simulink model "coneDetectionWithObjectDetectorBlock"  (R2025a)
settings: Solver=VariableStepAuto  StartTime=0.0  StopTime=50  RelTol=1e-3
undefined symbols (not defined in the file or in its folder): gray
libraries: visionanalysis x1, dspvision x1
settings Model: Creator=gracew  LastModifiedBy=lipingw
settings OptimizationCC: ReuseModelBlockBuffer=off
settings SFSimCC: SimTargetLang=C++  SimDLTargetLibrary=mkl-dnn
settings RTWCC: GPUComputeCapability=3.5

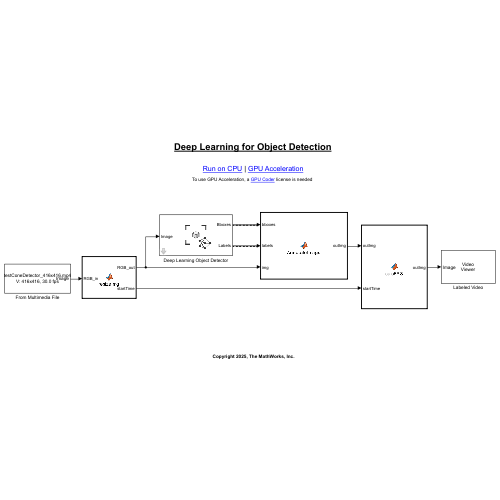
[thumbnail: Simulink's stored preview of the top-level diagram]
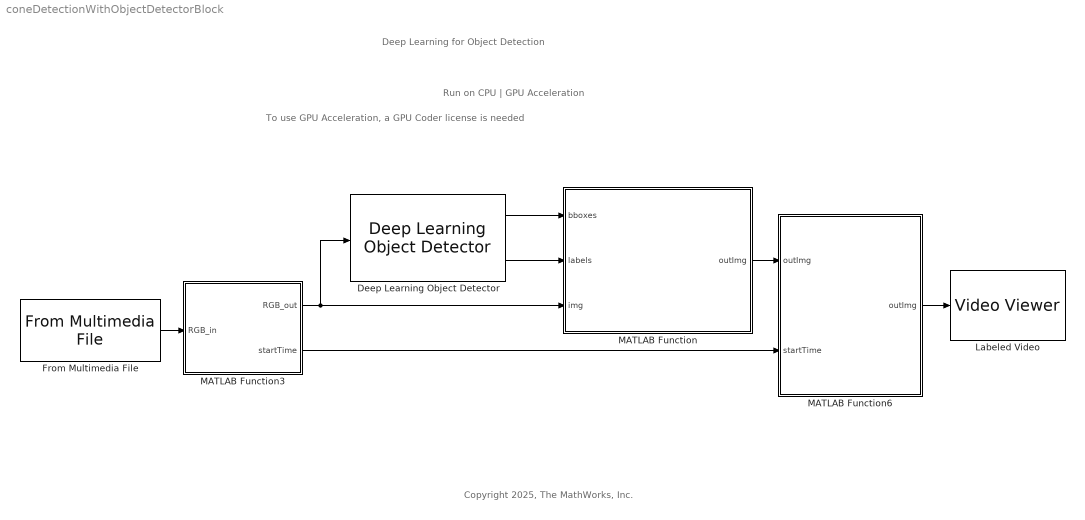
== system coneDetectionWithObjectDetectorBlock ==
  note: Deep Learning for Object Detection
  note: Run on CPU | GPU Acceleration
  note: To use GPU Acceleration, a GPU Coder license is needed
  note: Copyright 2025, The MathWorks, Inc.
  Deep Learning Object Detector : visionanalysis/Deep Learning Object Detector  Detector=Detector from MAT-file  DetectorFunction=untitled  DetectorFilePath=C:\MATLAB\cone-detection-using-deep-learning\yoloxConeDetector.mat  MaxDetections=500  Bboxes=on  Scores=off  UseROI=off  AutoResize=on  ROI=[1 1 100 100]  Threshold=0.5  NumStrongestRegions=2000  UseMinSize=off  MinSize=[1 1]  UseMaxSize=off  MaxSize=[50 50]  ForceInterpretedSim=off
  From Multimedia File : dspvision/From Multimedia File  inputFilename=C:\MATLAB\cone-detection-using-deep-learning\videos\testConeDetector_416x416.mp4  readRange=[1 Inf]  loop=on  numPlays=inf  outputStreams=Video only  videoDataType=uint8  audioDataType=int16  inheritSampleTime=on  userDefinedSampleTime=1  noAudioOutput=off  isIntensityVideo=off  fourcc=RGB  colorVideoFormat=One multidimensional signal  outputEOF=off  dataOrg=Column-major  audioFrameSize=1024  computeAudioFrameSize=off  outSamplingMode=Sample based
      settings: LibrarySourceBlock=visionsources/From Multimedia File
  Labeled Video : VideoViewer  colormapValue=gray(256)  FigPos=[5 717 1275 613]
  MATLAB Function : MATLAB Function  TreatAsAtomicUnit=on
  MATLAB Function3 : MATLAB Function  TreatAsAtomicUnit=on
  MATLAB Function6 : MATLAB Function  TreatAsAtomicUnit=on
  wires:
  Deep Learning Object Detector/1 -> MATLAB Function/1(bboxes)
  Deep Learning Object Detector/2 -> MATLAB Function/2(labels)
  MATLAB Function/1(outImg) -> MATLAB Function6/1("outImg ")
  MATLAB Function6/1(outImg) -> Labeled Video/1
  MATLAB Function3/1(RGB_out) -> MATLAB Function/3(img), Deep Learning Object Detector/1
  From Multimedia File/1 -> MATLAB Function3/1(RGB_in)
  MATLAB Function3/2(startTime) -> MATLAB Function6/2(startTime)

== matlab function coneDetectionWithObjectDetectorBlock/MATLAB Function ==
  data: bboxes input; labels input; outImg output; img input
function outImg = AnnotateImage(bboxes, labels, img)
    % Annotate detections in the image. 

    if ~isempty(bboxes)
        for i = 1:numel(labels)
            img = insertObjectAnnotation(img, "rectangle", bboxes(i, :), char(labels(i)));
        end
    end

    outImg = img;

end

== matlab function coneDetectionWithObjectDetectorBlock/MATLAB Function3 ==
  data: RGB_in input; RGB_out output; startTime output
function [RGB_out, startTime]  = resizeImg(RGB_in)
    RGB_out = imresize(RGB_in, [416,416]);
   
    currentTime = datetime;
    startTime = [currentTime.Year currentTime.Month currentTime.Day currentTime.Hour ...
    currentTime.Minute currentTime.Second];
end

== matlab function coneDetectionWithObjectDetectorBlock/MATLAB Function6 ==
  data: outImg input; outImg output; startTime input
function outImg  = calcFPS(outImg, startTime)
    finishTime = datetime;
    
    diffTime = seconds(finishTime-datetime(startTime));
    persistent count;
    if isempty(count)
        count = 0;
    end
    persistent fps;
    if isempty(fps)
        fps = 0;
    end
    fps = (count*fps + 1*(1/diffTime))/(count+1);

    count = count + 1;
    outImg = insertText(outImg, [10 80],['FPS : ' sprintf('%0.2f',fps) ], 'AnchorPoint','LeftBottom');
end
